simulink model "MRAC"  (R2021b)
settings: Solver=VariableStepAuto  StartTime=0.0  StopTime=TF  RelTol=1e-3
values from neighbouring files (symbols this model uses):
  Amplitude = 1/pi    (= 0.318309886184)    [Runner.m]
  Frequency = 1    [Runner.m]
  Phi = tanh(360/pi * q)    [AdaptiveLaws.m]    (also in Dynamics.m; Phi.m; u_ideal.m)
  q0 = .001    (= 0.001)    [Runner.m]
  q_ref0 = .001    (= 0.001)    [Runner.m]
  u0 = 0    [Runner.m]
undefined symbols (not defined in the file or in its folder): AdaptiveLaws, Dynamics, PitchRate
settings Model: Creator=maklenestrada  LastModifiedBy=maklenestrada

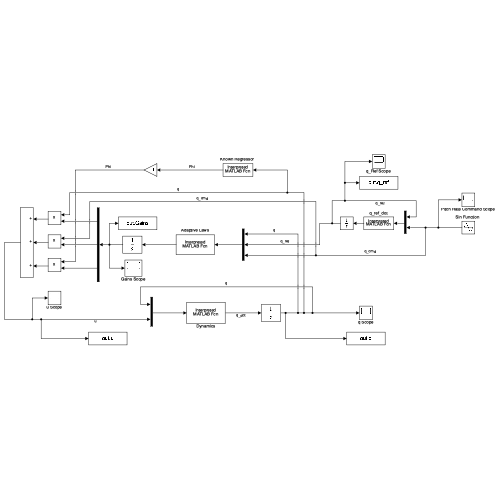
[thumbnail: Simulink's stored preview of the top-level diagram]
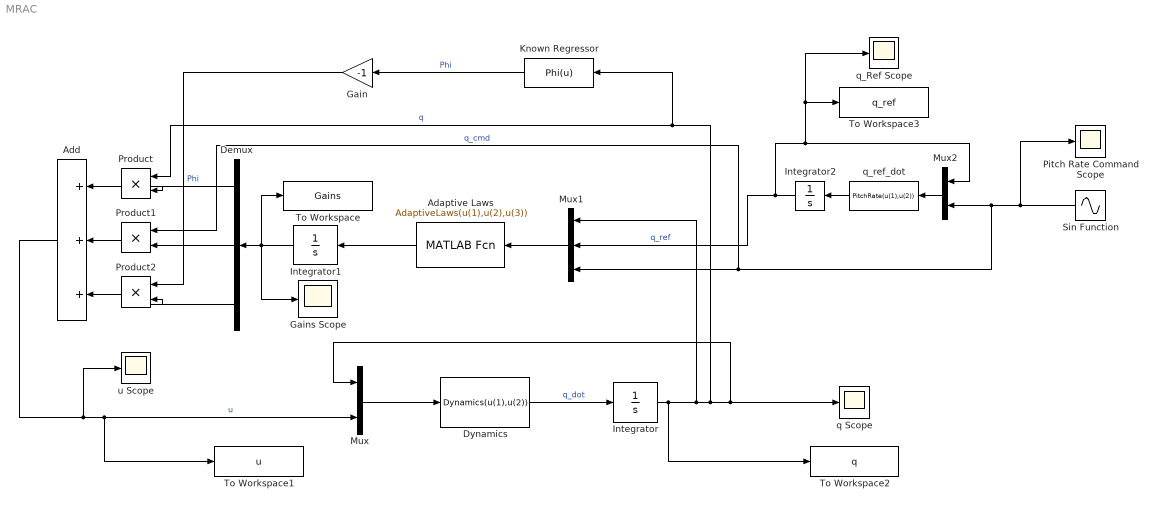
== system MRAC ==
  Adaptive Laws : MATLABFcn  MATLABFcn=AdaptiveLaws(u(1),u(2),u(3))  OutputDimensions=3
  Add : Sum  Inputs=+++
  Demux : Demux  Outputs=3
  Dynamics : MATLABFcn  MATLABFcn=Dynamics(u(1),u(2))
  Gain : Gain  Gain=-1
  Gains Scope : Scope
  Integrator : Integrator  InitialCondition=q0
  Integrator1 : Integrator  InitialCondition=u0
  Integrator2 : Integrator  InitialCondition=q_ref0
  "Known Regressor " : MATLABFcn  MATLABFcn=Phi(u)
  Mux : Mux  Inputs=2
  Mux1 : Mux  Inputs=3
  Mux2 : Mux  Inputs=2
  Pitch Rate Command Scope : Scope
  Product : Product
  Product1 : Product
  Product2 : Product
  "Sin Function " : Sin  Amplitude=Amplitude  Frequency=Frequency  SampleTime=0
  To Workspace : ToWorkspace  VariableName=Gains  SaveFormat=Timeseries  SampleTime=-1
  To Workspace1 : ToWorkspace  VariableName=u  SaveFormat=Timeseries  SampleTime=-1
  To Workspace2 : ToWorkspace  VariableName=q  SaveFormat=Timeseries  SampleTime=-1
  To Workspace3 : ToWorkspace  VariableName=q_ref  SaveFormat=Timeseries  SampleTime=-1
  q Scope : Scope
  q_Ref Scope : Scope
  q_ref_dot : MATLABFcn  MATLABFcn=PitchRate(u(1),u(2))
  u Scope : Scope
  wires:
  Dynamics/1 -> Integrator/1  "q_dot"
  Integrator/1 -> q Scope/1, Mux/1, "Known Regressor "/1, Product/1, Mux1/1, To Workspace2/1  "q"
  Adaptive Laws/1 -> Integrator1/1
  Integrator1/1 -> Gains Scope/1, To Workspace/1, Demux/1
  Demux/1 -> Product/2
  Demux/2 -> Product1/2
  Demux/3 -> Product2/2
  "Sin Function "/1 -> Pitch Rate Command Scope/1, Product1/1, Mux1/3, Mux2/2  "q_cmd"
  Mux1/1 -> Adaptive Laws/1
  q_ref_dot/1 -> Integrator2/1
  Integrator2/1 -> q_Ref Scope/1, To Workspace3/1, Mux2/1, Mux1/2  "q_ref"
  "Known Regressor "/1 -> Gain/1  "Phi"
  Gain/1 -> Product2/1  "Phi"
  Product/1 -> Add/1
  Product1/1 -> Add/2
  Product2/1 -> Add/3
  Add/1 -> u Scope/1, To Workspace1/1, Mux/2  "u"
  Mux/1 -> Dynamics/1
  Mux2/1 -> q_ref_dot/1
